simulink model "BasicQuadrotorControl_interface"  (R2014b)
settings: Solver=FixedStepDiscrete  StartTime=0.0  StopTime=inf  RelTol=1e-3
PostLoadFcn:
  | Ts = 1/1e3;  % Run ARM process at 1KHz
  | READ_CMD = uint16(bin2dec('1000000000000000'));
  | DATA_FORMAT =  uint16(hex2dec('3108'));
  | POWER_ON =  uint16(hex2dec('2D08'));
  | % you can add any number of initialization commands here
  | INIT_CMDS = [POWER_ON, POWER_ON, POWER_ON, DATA_FORMAT, DATA_FORMAT, DATA_FORMAT,READ_CMD];
undefined symbols (not defined in the file): AXI4, Lite
libraries: axiinterfacelib x10, simulink x3
settings Model: SimulationMode=external  Creator=bsoheili  LastModifiedBy=dlwalter
settings SolverCC: PositivePriorityOrder=on
settings DataIOCC: SaveOutput=off  SaveTime=off
settings OptimizationCC: OptimizeModelRefInitCode=on  LifeSpan=1  MaxStackSize=64
settings DebuggingCC: UnderspecifiedInitializationDetection=Classic  MergeDetectMultiDrivingBlocksExec=none
settings HardwareCC: ProdLargestAtomicInteger=Long  ProdLargestAtomicFloat=Double  ProdEndianess=LittleEndian  ProdHWDeviceType=ARM Compatible->ARM Cortex  TargetLargestAtomicInteger=Long  TargetLargestAtomicFloat=Double  TargetIntDivRoundTo=Zero  TargetEndianess=LittleEndian  TargetHWDeviceType=ARMCortex  ProdEqTarget=off
settings RTWCC: SystemTargetFile=ert.tlc  TLCOptions=-aInlineSetEventsForThisBaseRateFcn=TLC_FALSE -aSuppressMultiTaskScheduler=TLC_FALSE  TemplateMakefile=ert_default_tmf  Description=Embedded Coder  ProcessScript=idelink_ert_make_rtw_hook  Toolchain=Xilinx ISE Design Suite 14.4
settings CodeAppCC: IgnoreCustomStorageClasses=off
settings ERTTargetCC: ParMdlRefBuildCompliant=off  GeneratePreprocessorConditionals=Disable all  CPPClassGenCompliant=off  ExtMode=on  ExtModeMexArgs='172.30.27.249'

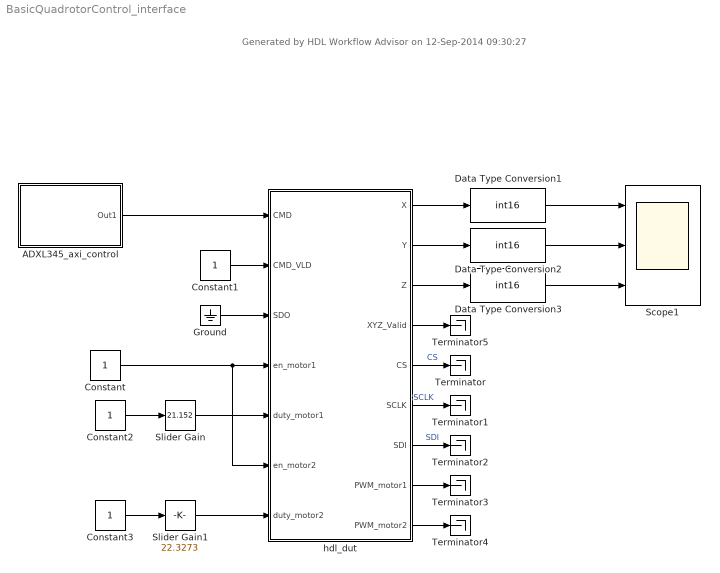
== system BasicQuadrotorControl_interface ==
  note: Generated by HDL Workflow Advisor on 12-Sep-2014 09:30:27
  ADXL345_axi_control : Subsystem
  Constant : Constant  OutDataTypeStr=boolean  SampleTime=-1
  Constant1 : Constant  SampleTime=-1
  Constant2 : Constant  OutDataTypeStr=uint8  SampleTime=-1
  Constant3 : Constant  OutDataTypeStr=uint8  SampleTime=-1
  Data Type Conversion1 : DataTypeConversion  OutDataTypeStr=int16
  Data Type Conversion2 : DataTypeConversion  OutDataTypeStr=int16
  Data Type Conversion3 : DataTypeConversion  OutDataTypeStr=int16
  Ground : Ground
  Scope1 : Scope  NumInputPorts=3
      settings: TickLabels=on  TimeRange=5  YMin=-500~-500~1000  YMax=2000~1500~8000  SaveName=ScopeData2
  Slider Gain : simulink/Math Operations/Slider Gain  low=0  gain=21.152  high=255
  Slider Gain1 : simulink/Math Operations/Slider Gain  low=0  gain=22.3273  high=255
  Terminator{,1..5} (6 alike) : Terminator
  hdl_dut : Subsystem  TreatAsAtomicUnit=on  mask(AXI4-Lite/AXI4 Interface){}
      mask help:
      | This is an automatically generated subsystem block.
      | This contains the AXI4-Lite/AXI4 interface which communicates with the basicquadrotorcontrol_hdl_dut_pcore IPCore generated from BasicQuadrotorControl/hdl_dut subsystem.
      mask Display: disp(sprintf('Xilinx Zynq \nAXI4-Lite/AXI4 Interface'));
  wires:
  Ground/1 -> hdl_dut/3(SDO)
  hdl_dut/7(SDI) -> Terminator2/1  "SDI"
  hdl_dut/6(SCLK) -> Terminator1/1  "SCLK"
  hdl_dut/5(CS) -> Terminator/1  "CS"
  Constant1/1 -> hdl_dut/2(CMD_VLD)
  hdl_dut/1(X) -> Data Type Conversion1/1
  hdl_dut/3(Z) -> Data Type Conversion3/1
  hdl_dut/2(Y) -> Data Type Conversion2/1
  Data Type Conversion1/1 -> Scope1/1
  Data Type Conversion2/1 -> Scope1/2
  Data Type Conversion3/1 -> Scope1/3
  hdl_dut/8(PWM_motor1) -> Terminator3/1
  hdl_dut/9(PWM_motor2) -> Terminator4/1
  ADXL345_axi_control/1(Out1) -> hdl_dut/1(CMD)
  Constant/1 -> hdl_dut/6(en_motor2), hdl_dut/4(en_motor1)
  Constant2/1 -> Slider Gain/1
  Slider Gain/1 -> hdl_dut/5(duty_motor1)
  Constant3/1 -> Slider Gain1/1
  Slider Gain1/1 -> hdl_dut/7(duty_motor2)
  hdl_dut/4(XYZ_Valid) -> Terminator5/1

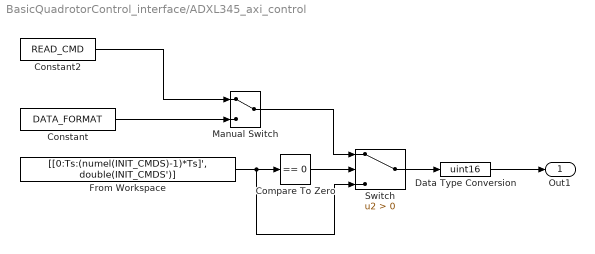
== system BasicQuadrotorControl_interface/ADXL345_axi_control ==
  Compare To Zero : simulink/Logic and Bit Operations/Compare To Zero  relop===  OutDataTypeStr=boolean
  Constant : Constant  Value=DATA_FORMAT  SampleTime=-1
  Constant2 : Constant  Value=READ_CMD  SampleTime=-1
  Data Type Conversion : DataTypeConversion  OutDataTypeStr=uint16
  From Workspace : FromWorkspace  VariableName=[[0:Ts:(numel(INIT_CMDS)-1)*Ts]', double(INIT_CMDS')]  SampleTime=Ts  Interpolate=off  OutputAfterFinalValue=Setting to zero
  Manual Switch : ManualSwitch
  Switch : Switch  Criteria=u2 > Threshold
  Out1 : Outport
  wires:
  Data Type Conversion/1 -> Out1/1
  From Workspace/1 -> Switch/3, Compare To Zero/1
  Switch/1 -> Data Type Conversion/1
  Constant/1 -> Manual Switch/2
  Compare To Zero/1 -> Switch/2
  Constant2/1 -> Manual Switch/1
  Manual Switch/1 -> Switch/1

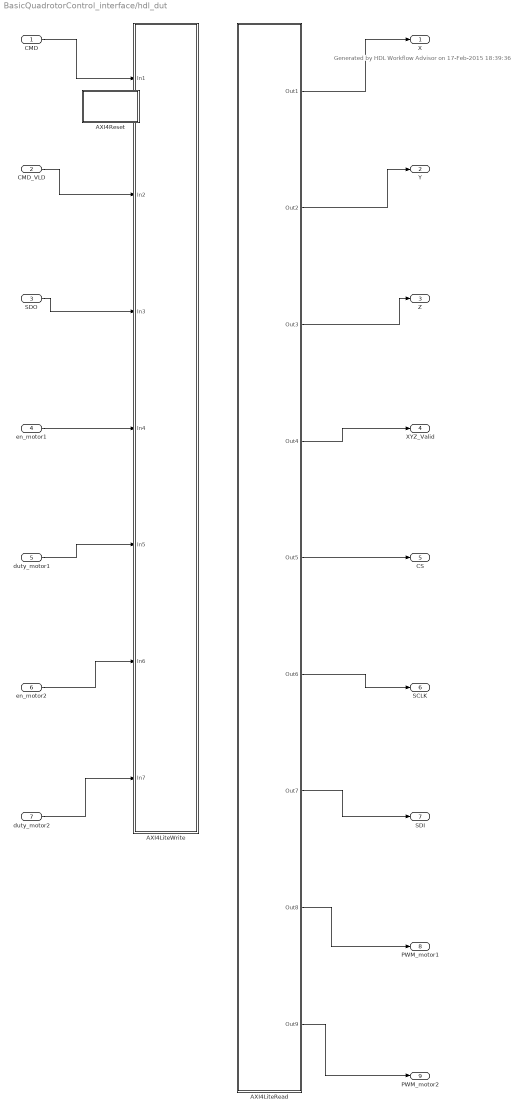
== system BasicQuadrotorControl_interface/hdl_dut ==
  note: Generated by HDL Workflow Advisor on 17-Feb-2015 18:39:36
  CMD : Inport
  CMD_VLD : Inport  Port=2
  SDO : Inport  Port=3
  en_motor1 : Inport  Port=4
  duty_motor1 : Inport  Port=5
  en_motor2 : Inport  Port=6
  duty_motor2 : Inport  Port=7
  AXI4LiteRead : Subsystem  Priority=10
  AXI4LiteWrite : Subsystem  Priority=1
  AXI4Reset : Subsystem  mask(System Initialize){ShowInLibBrowser=0}
      mask prompts: ShowInLibBrowser "Simulink:masks:CustCodeMaskParam1_MP"
      settings: CopyFcn=cccopyfcn(gcb)  OpenFcn=ccopenfcn('System Initialize Function')
      mask Help: eval('feval(''rtwprivate'',''rtwhelpview'',''rtw_sys_initialize_block'')');
      mask Display: disp('System\nInitialize');
  X : Outport
  Y : Outport  Port=2
  Z : Outport  Port=3
  XYZ_Valid : Outport  Port=4
  CS : Outport  Port=5
  SCLK : Outport  Port=6
  SDI : Outport  Port=7
  PWM_motor1 : Outport  Port=8  OutDataTypeStr=boolean
  PWM_motor2 : Outport  Port=9  OutDataTypeStr=boolean
  wires:
  CMD/1 -> AXI4LiteWrite/1(In1)
  CMD_VLD/1 -> AXI4LiteWrite/2(In2)
  SDO/1 -> AXI4LiteWrite/3(In3)
  en_motor1/1 -> AXI4LiteWrite/4(In4)
  duty_motor1/1 -> AXI4LiteWrite/5(In5)
  en_motor2/1 -> AXI4LiteWrite/6(In6)
  duty_motor2/1 -> AXI4LiteWrite/7(In7)
  AXI4LiteRead/1(Out1) -> X/1
  AXI4LiteRead/2(Out2) -> Y/1
  AXI4LiteRead/3(Out3) -> Z/1
  AXI4LiteRead/4(Out4) -> XYZ_Valid/1
  AXI4LiteRead/5(Out5) -> CS/1
  AXI4LiteRead/6(Out6) -> SCLK/1
  AXI4LiteRead/7(Out7) -> SDI/1
  AXI4LiteRead/8(Out8) -> PWM_motor1/1
  AXI4LiteRead/9(Out9) -> PWM_motor2/1

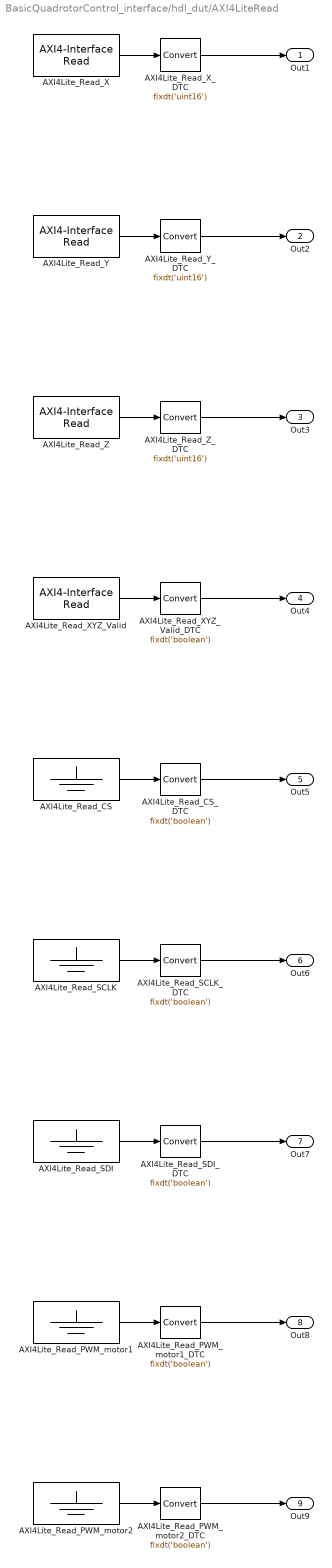
== system BasicQuadrotorControl_interface/hdl_dut/AXI4LiteRead ==
  AXI4Lite_Read_CS : Ground
  AXI4Lite_Read_CS_DTC : DataTypeConversion  OutDataTypeStr=fixdt('boolean')  ConvertRealWorld=Stored Integer (SI)
  AXI4Lite_Read_PWM_motor1 : Ground
  AXI4Lite_Read_PWM_motor1_DTC : DataTypeConversion  OutDataTypeStr=fixdt('boolean')  ConvertRealWorld=Stored Integer (SI)
  AXI4Lite_Read_PWM_motor2 : Ground
  AXI4Lite_Read_PWM_motor2_DTC : DataTypeConversion  OutDataTypeStr=fixdt('boolean')  ConvertRealWorld=Stored Integer (SI)
  AXI4Lite_Read_SCLK : Ground
  AXI4Lite_Read_SCLK_DTC : DataTypeConversion  OutDataTypeStr=fixdt('boolean')  ConvertRealWorld=Stored Integer (SI)
  AXI4Lite_Read_SDI : Ground
  AXI4Lite_Read_SDI_DTC : DataTypeConversion  OutDataTypeStr=fixdt('boolean')  ConvertRealWorld=Stored Integer (SI)
  AXI4Lite_Read_X : axiinterfacelib/AXI4-Interface Read  Priority=2  AXIInterfaceType=AXI4-Lite  DeviceName=/dev/mwipcore  RegisterOffset=hex2dec('108')  DataType=uint32  DataLength=4096  SampleTime=-1  blockPlatform=ZYNQ  SimulateUsing=Interpreted Execution
  AXI4Lite_Read_XYZ_Valid : axiinterfacelib/AXI4-Interface Read  Priority=5  AXIInterfaceType=AXI4-Lite  DeviceName=/dev/mwipcore  RegisterOffset=hex2dec('114')  DataType=uint32  DataLength=4096  SampleTime=-1  blockPlatform=ZYNQ  SimulateUsing=Interpreted Execution
  AXI4Lite_Read_XYZ_Valid_DTC : DataTypeConversion  OutDataTypeStr=fixdt('boolean')  ConvertRealWorld=Stored Integer (SI)
  AXI4Lite_Read_X_DTC : DataTypeConversion  OutDataTypeStr=fixdt('uint16')  ConvertRealWorld=Stored Integer (SI)
  AXI4Lite_Read_Y : axiinterfacelib/AXI4-Interface Read  Priority=3  AXIInterfaceType=AXI4-Lite  DeviceName=/dev/mwipcore  RegisterOffset=hex2dec('10C')  DataType=uint32  DataLength=4096  SampleTime=-1  blockPlatform=ZYNQ  SimulateUsing=Interpreted Execution
  AXI4Lite_Read_Y_DTC : DataTypeConversion  OutDataTypeStr=fixdt('uint16')  ConvertRealWorld=Stored Integer (SI)
  AXI4Lite_Read_Z : axiinterfacelib/AXI4-Interface Read  Priority=4  AXIInterfaceType=AXI4-Lite  DeviceName=/dev/mwipcore  RegisterOffset=hex2dec('110')  DataType=uint32  DataLength=4096  SampleTime=-1  blockPlatform=ZYNQ  SimulateUsing=Interpreted Execution
  AXI4Lite_Read_Z_DTC : DataTypeConversion  OutDataTypeStr=fixdt('uint16')  ConvertRealWorld=Stored Integer (SI)
  Out1 : Outport
  Out2 : Outport  Port=2
  Out3 : Outport  Port=3
  Out4 : Outport  Port=4
  Out5 : Outport  Port=5
  Out6 : Outport  Port=6
  Out7 : Outport  Port=7
  Out8 : Outport  Port=8
  Out9 : Outport  Port=9
  wires:
  AXI4Lite_Read_Y_DTC/1 -> Out2/1
  AXI4Lite_Read_Y/1 -> AXI4Lite_Read_Y_DTC/1
  AXI4Lite_Read_X_DTC/1 -> Out1/1
  AXI4Lite_Read_X/1 -> AXI4Lite_Read_X_DTC/1
  AXI4Lite_Read_Z_DTC/1 -> Out3/1
  AXI4Lite_Read_Z/1 -> AXI4Lite_Read_Z_DTC/1
  AXI4Lite_Read_PWM_motor1_DTC/1 -> Out8/1
  AXI4Lite_Read_SCLK_DTC/1 -> Out6/1
  AXI4Lite_Read_XYZ_Valid_DTC/1 -> Out4/1
  AXI4Lite_Read_SDI_DTC/1 -> Out7/1
  AXI4Lite_Read_SDI/1 -> AXI4Lite_Read_SDI_DTC/1
  AXI4Lite_Read_PWM_motor2/1 -> AXI4Lite_Read_PWM_motor2_DTC/1
  AXI4Lite_Read_SCLK/1 -> AXI4Lite_Read_SCLK_DTC/1
  AXI4Lite_Read_PWM_motor2_DTC/1 -> Out9/1
  AXI4Lite_Read_XYZ_Valid/1 -> AXI4Lite_Read_XYZ_Valid_DTC/1
  AXI4Lite_Read_PWM_motor1/1 -> AXI4Lite_Read_PWM_motor1_DTC/1
  AXI4Lite_Read_CS_DTC/1 -> Out5/1
  AXI4Lite_Read_CS/1 -> AXI4Lite_Read_CS_DTC/1

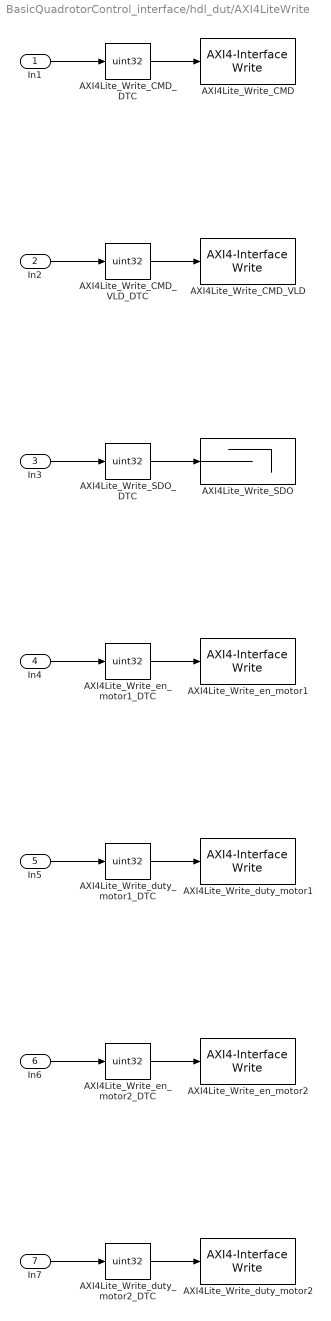
== system BasicQuadrotorControl_interface/hdl_dut/AXI4LiteWrite ==
  In1 : Inport
  In2 : Inport  Port=2
  In3 : Inport  Port=3
  In4 : Inport  Port=4
  In5 : Inport  Port=5
  In6 : Inport  Port=6
  In7 : Inport  Port=7
  AXI4Lite_Write_CMD : axiinterfacelib/AXI4-Interface Write  Priority=1  AXIInterfaceType=AXI4-Lite  DeviceName=/dev/mwipcore  RegisterOffset=hex2dec('100')  blockPlatform=ZYNQ  SimulateUsing=Interpreted execution
  AXI4Lite_Write_CMD_DTC : DataTypeConversion  OutDataTypeStr=uint32  ConvertRealWorld=Stored Integer (SI)
  AXI4Lite_Write_CMD_VLD : axiinterfacelib/AXI4-Interface Write  Priority=2  AXIInterfaceType=AXI4-Lite  DeviceName=/dev/mwipcore  RegisterOffset=hex2dec('104')  blockPlatform=ZYNQ  SimulateUsing=Interpreted execution
  AXI4Lite_Write_CMD_VLD_DTC : DataTypeConversion  OutDataTypeStr=uint32  ConvertRealWorld=Stored Integer (SI)
  AXI4Lite_Write_SDO : Terminator
  AXI4Lite_Write_SDO_DTC : DataTypeConversion  OutDataTypeStr=uint32  ConvertRealWorld=Stored Integer (SI)
  AXI4Lite_Write_duty_motor1 : axiinterfacelib/AXI4-Interface Write  Priority=5  AXIInterfaceType=AXI4-Lite  DeviceName=/dev/mwipcore  RegisterOffset=hex2dec('11C')  blockPlatform=ZYNQ  SimulateUsing=Interpreted execution
  AXI4Lite_Write_duty_motor1_DTC : DataTypeConversion  OutDataTypeStr=uint32  ConvertRealWorld=Stored Integer (SI)
  AXI4Lite_Write_duty_motor2 : axiinterfacelib/AXI4-Interface Write  Priority=7  AXIInterfaceType=AXI4-Lite  DeviceName=/dev/mwipcore  RegisterOffset=hex2dec('124')  blockPlatform=ZYNQ  SimulateUsing=Interpreted execution
  AXI4Lite_Write_duty_motor2_DTC : DataTypeConversion  OutDataTypeStr=uint32  ConvertRealWorld=Stored Integer (SI)
  AXI4Lite_Write_en_motor1 : axiinterfacelib/AXI4-Interface Write  Priority=4  AXIInterfaceType=AXI4-Lite  DeviceName=/dev/mwipcore  RegisterOffset=hex2dec('118')  blockPlatform=ZYNQ  SimulateUsing=Interpreted execution
  AXI4Lite_Write_en_motor1_DTC : DataTypeConversion  OutDataTypeStr=uint32  ConvertRealWorld=Stored Integer (SI)
  AXI4Lite_Write_en_motor2 : axiinterfacelib/AXI4-Interface Write  Priority=6  AXIInterfaceType=AXI4-Lite  DeviceName=/dev/mwipcore  RegisterOffset=hex2dec('120')  blockPlatform=ZYNQ  SimulateUsing=Interpreted execution
  AXI4Lite_Write_en_motor2_DTC : DataTypeConversion  OutDataTypeStr=uint32  ConvertRealWorld=Stored Integer (SI)
  wires:
  In1/1 -> AXI4Lite_Write_CMD_DTC/1
  AXI4Lite_Write_CMD_DTC/1 -> AXI4Lite_Write_CMD/1
  In2/1 -> AXI4Lite_Write_CMD_VLD_DTC/1
  In4/1 -> AXI4Lite_Write_en_motor1_DTC/1
  In3/1 -> AXI4Lite_Write_SDO_DTC/1
  In5/1 -> AXI4Lite_Write_duty_motor1_DTC/1
  AXI4Lite_Write_duty_motor1_DTC/1 -> AXI4Lite_Write_duty_motor1/1
  AXI4Lite_Write_en_motor1_DTC/1 -> AXI4Lite_Write_en_motor1/1
  AXI4Lite_Write_CMD_VLD_DTC/1 -> AXI4Lite_Write_CMD_VLD/1
  AXI4Lite_Write_SDO_DTC/1 -> AXI4Lite_Write_SDO/1
  In7/1 -> AXI4Lite_Write_duty_motor2_DTC/1
  In6/1 -> AXI4Lite_Write_en_motor2_DTC/1
  AXI4Lite_Write_en_motor2_DTC/1 -> AXI4Lite_Write_en_motor2/1
  AXI4Lite_Write_duty_motor2_DTC/1 -> AXI4Lite_Write_duty_motor2/1

== system BasicQuadrotorControl_interface/hdl_dut/AXI4Reset ==
